simulink model "02-07-2026"  (R2025b)
settings: Solver=ode5  StartTime=0.0  StopTime=150  FixedStep=1/3200  RelTol=1e-3
model workspace (MAT data in the model file):
  mass = 7
  radius = 333
libraries: simulink x5, simulink_extras x4, eeGeneralControl x2
settings Model: Creator=Fabian  LastModifiedBy=fabia

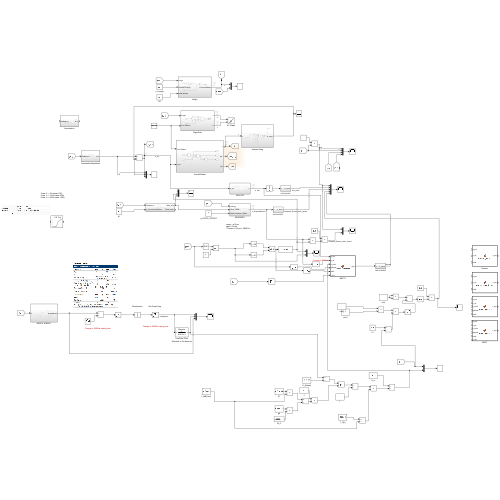
[thumbnail: Simulink's stored preview of the top-level diagram]
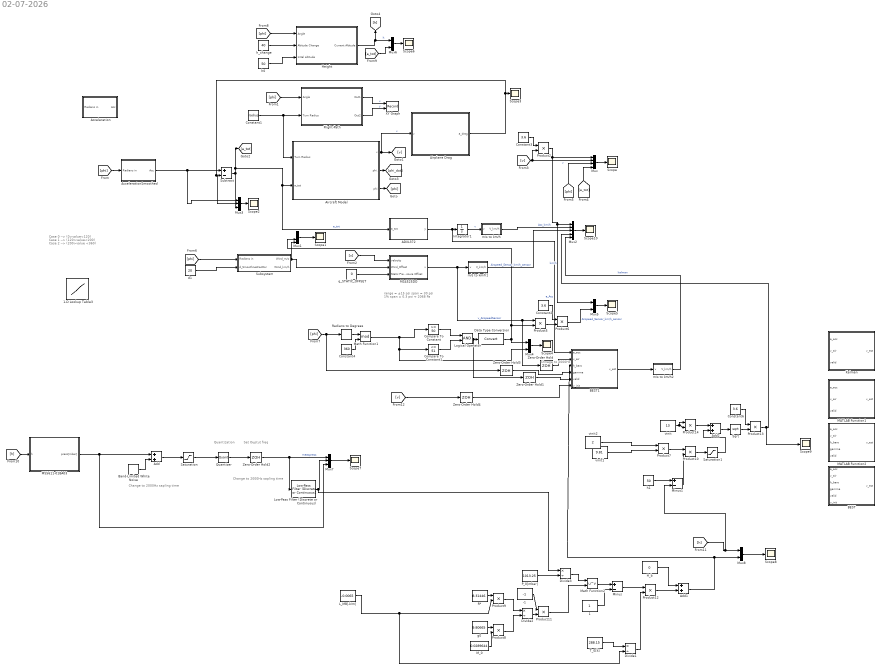
== system 02-07-2026 ==
  note: Change to 2000Hz sapling time
  note: Chnage to 2000Hz
  note: range = ±15 psi
      | span = 30 psi
      | 1% span = 0.3 psi ≈ 2068 Pa
  note: Case 0 --> (0>value<120)
      | Case 1 --> (120>value<200)
      | Case 2 --> (200>value <360)
  note: Set Ouptut freq
  note: Quantization
  note: Change to 2000Hz sapling time
  -1 : Constant  Value=-1
  1 : Constant
  1-D Lookup Table3 : Lookup_n-D  NumberOfTableDimensions=1  BreakpointsForDimension1=[0 110 130 190 210 360]  Table=[30 20 30 60 90 120]  InternalRulePriority=Speed  RndMeth=Simplest
  ADXL372 : Subsystem
  Acceleration : Subsystem
  AccelerationSmoothed : Subsystem
  Add : Sum
  Add1 : Sum
  Add2 : Sum
  Aircraft Model : Subsystem
  Airplane Drag : Subsystem
  BEST : MATLAB Function  TreatAsAtomicUnit=on
  BEST1 : MATLAB Function  TreatAsAtomicUnit=on
  Band-Limited White Noise : simulink/Sources/Band-Limited White Noise  Cov=(0.065)^2 * (1/2000)  Ts=1/3200  seed=[23341]
  Compare To Constant : simulink/Logic and Bit Operations/Compare To Constant  relop=>=  const=50  OutDataTypeStr=boolean
  Compare To Constant1 : simulink/Logic and Bit Operations/Compare To Constant  relop=<=  const=51  OutDataTypeStr=boolean
  Constant1 : Constant  Value=radius
  Constant2 : Constant  Value=3.6
  Constant3 : Constant  Value=3.6
  Constant4 : Constant  Value=360
  Constant6 : Constant  Value=3.6
  Data Type Conversion : DataTypeConversion  SaturateOnIntegerOverflow=off  RndMeth=Floor
  Divide1 : Product  Inputs=*/
  Divide2 : Product  Inputs=*/
  Divide3 : Product  Inputs=*/
  Flight-Path : Subsystem
  H_b : Constant  Value=0
  Height : Subsystem
  Integrator1 : Integrator  InitialCondition=13
  Kalman : MATLAB Function  TreatAsAtomicUnit=on
  L_MB[-k/m] : Constant  Value=-0.0065
  Logical Operator : Logic  AllPortsSameDT=off  OutDataTypeStr=fixdt(1,16)
  Low-Pass Filter (Discrete or Continuous) : eeGeneralControl/Low-Pass Filter (Discrete or Continuous)  K=1  T=0.021  B=inf  A=-inf  init_option=Inherited from block input  x0=0  Ts=-1
  MATLAB Function1 : MATLAB Function  TreatAsAtomicUnit=on
  MATLAB Function2 : MATLAB Function  TreatAsAtomicUnit=on
  MS4525DO : Subsystem
  "MS5611-01BA03 " : Subsystem
  M_0 : Constant  Value=0.0289644
  Math Function1 : Math  Operator=mod
  Math Function2 : Math  Operator=pow
  Minus : Sum  Inputs=+-
  Minus1 : Sum  Inputs=+-
  Mux : Mux
  Mux1 : Mux
  Mux2 : Mux  Inputs=5
  Mux3 : Mux  Inputs=3
  Mux{4..6,8} (4 alike) : Mux  Inputs=2
  Mux7 : Mux  Inputs=3
  P_0[mbar] : Constant  Value=1013.25
  Product{2,5..14} (11 alike) : Product
  Quantizer : Quantizer  QuantizationInterval=(1200-10)/(2^24)
  R* : Constant  Value=8.31446
  Radians to Degrees : simulink_extras/Transformations/Radians to Degrees
  Saturation : Saturate  UpperLimit=1200  LowerLimit=10
  Saturation1 : Saturate  UpperLimit=inf  LowerLimit=0.1
  Scope{,1..10} (11 alike) : Scope
      Scope settings: ActiveDisplayYMinimum=-135.5578997044986  ActiveDisplayYMaximum=1137.6664983393619
      Scope1 settings: ActiveDisplayYMinimum=-14.999999155382156  ActiveDisplayYMaximum=134.99999239843945  DataLoggingVariableName=ScopeData2
      Scope10 settings: ActiveDisplayYMinimum=-69.890870936461468  ActiveDisplayYMaximum=1097.0178384281537  DataLoggingVariableName=ScopeData11
      Scope2 settings: ActiveDisplayYMinimum=-39.208466924616559  ActiveDisplayYMaximum=63.33696033694325  DataLoggingVariableName=ScopeData3
      Scope3 settings: ActiveDisplayYMinimum=-3.5843354434410593  ActiveDisplayYMaximum=33.486381490969542  DataLoggingVariableName=ScopeData6
      Scope4 settings: ActiveDisplayYMinimum=-31.576019805247327  ActiveDisplayYMaximum=399.38392905519919  DataLoggingVariableName=ScopeData9
      Scope5 settings: ActiveDisplayYMinimum=189.29544667943134  ActiveDisplayYMaximum=704.92209117020684  DataLoggingVariableName=ScopeData12
      Scope6 settings: ActiveDisplayYMinimum=-31.394100237137991  ActiveDisplayYMaximum=92.400581276019  DataLoggingVariableName=ScopeData13
      Scope7 settings: ActiveDisplayYMinimum=1004.7404966647082  ActiveDisplayYMaximum=1013.7440475042908  DataLoggingVariableName=ScopeData14
      Scope8 settings: ActiveDisplayYMinimum=85.0381751510035  ActiveDisplayYMaximum=91.4462483318631  DataLoggingVariableName=ScopeData15
      Scope9 settings: ActiveDisplayYMinimum=38.767930934422381  ActiveDisplayYMaximum=119.22706265224174  DataLoggingVariableName=ScopeData16
  Sqrt : Sqrt
  Subsystem : Subsystem
  Subtract : Sum  Inputs=+-
  T_0[k] : Constant  Value=288.15
  XY Graph : Record  NumPorts=2.0  FileSettingsInternal="{\"entries\":[{\"content\":{\"excelSettings\":{\"content\":{},\"type\":\"Streamout.ExcelSettings\"},\"parquetSettings\":{\"content\":{},\"type\":\"Streamout.ParquetSettings\"}},\"type\":\"Streamout.FileSettingStorage\",\"uuid\":\"\"}],\"packageUris\":[\"http:\\/\\/schema.mathworks.com\\/mf0\\/streamout_blocks\\/R2020a\"],\"version\":\"1.0\"}"  FrameSettings=[0, 0]  Layout=[1 1]  SignalsInternal="{\"entries\":[{\"content\":{\"signals\":[{\"content\":{\"blockPath\":[],\"dimensions\":[1],\"domain\":\"\",\"lineColor\":\"#a2142f\",\"plots\":[ 1 ],\"port\":1,\"sid\":[\"\"],\"signalID\":1,\"signalName\":\"x\"},\"type\":\"RecordBlkView.Signal\",\"uuid\":\"\"},{\"content\":{\"blockPath\":[],\"dimensions\":[1],\"domain\":\"\",\"lineColor\":\"#139fff\",\"plots\":[ 1 ],\"port\":2,\"sid\":[\"\"],\"signalID\":2,\"signalName\":\"y\"},\"type\":\"RecordBlkView.Signal\",\"uuid\":\"\"}]},\"type\":\"RecordBlkView.InputSignals\",\"uuid\":\"\"}],\"packageUris\":[\"http:\\/\\/schema.mathworks.com\\/mf0\\/streamout_blocks\\/R2020a\"],\"version\":\"1.0\"}"  VisualizationBindings="{\"xyplotplugin\":{\"info\":[{\"series\":[{\"bindingParametersList\":[{\"parameter\":\"X-Axis\",\"signalID\":1,\"signalName\":\"x\"},{\"parameter\":\"Y-Axis\",\"signalID\":2,\"signalName\":\"y\"}],\"seriesID\":0}],\"subplotID\":1}]}}"  CompatibilityTag=XY
  Zero-Order Hold{,1..4} (5 alike) : ZeroOrderHold  SampleTime=1/3200
  d1 : Constant  Value=20
  g0 : Constant  Value=9.80665
  h0 : Constant  Value=50
  h1 : Constant  Value=50
  h_change : Constant  Value=40
  m/s to km/h : Subsystem
  m/s to km/h1 : Subsystem
  m/s to km/h2 : Subsystem
  q_STATIC_OFFSET : Constant  Value=0
  vinit : Constant  Value=13
  vinit1 : Constant  Value=9.81
  vinit2 : Constant  Value=2
  wires:
  Subtract/1 -> [a_tot], ADXL372/1(a_tot), Aircraft Model/2(a_tot), Mux3/3  "a_tot"
  Constant1/1 -> Flight-Path/2(Turn Radius), Aircraft Model/1(Turn Radius)
  Product2/1 -> Mux2/1, Mux5/1, Mux/1  "km/h"
  Mux2/1 -> Scope10/1
  ADXL372/1(y) -> BEST1/1(a_acc), Integrator1/1  "a_Acc"
  [phi] -> AccelerationSmoothed/1(Radians in)
  m/s to km/h1/1(V_km/h) -> Mux2/3  "Airspeed_Sensor_km/h_sensor"
  [v] -> MS4525DO/1(velocity)
  q_STATIC_OFFSET/1 -> MS4525DO/3(Static Pressure Offset)
  MS4525DO/1(v) -> m/s to km/h1/1(v), Zero-Order Hold/1, Product5/1  "v_AirspeedSensor"
  [phi] -> Flight-Path/1(Angle)
  Flight-Path/1(Out1) -> XY Graph/1  "x"
  Flight-Path/2(Out2) -> XY Graph/2  "y"
  [v] -> Product2/2, Mux/2  "v"
  [a_tot] -> Mux/4
  [phi] -> Mux/3
  Aircraft Model/1(v) -> Airplane Drag/1(v), [v]  "v"
  Aircraft Model/2(phi.) -> [phi_dot]
  Aircraft Model/3(phi) -> [phi]
  Constant3/1 -> Product2/1
  Mux/1 -> Scope/1
  Mux1/1 -> Scope1/1
  Mux3/1 -> Scope2/1
  [phi] -> Subsystem/1(Radians in)
  d1/1 -> Subsystem/2(d_SmoothnesFacttor)
  Subsystem/1(Wind_m/s) -> Mux1/4, MS4525DO/2(Wind_Offset)
  AccelerationSmoothed/1(Acc) -> Mux3/1, Subtract/1
  [phi] -> Zero-Order Hold3/1, Radians to Degrees/1
  Radians to Degrees/1 -> Math Function1/1
  Constant4/1 -> Math Function1/2
  Math Function1/1 -> Compare To Constant/1, Compare To Constant1/1, Mux4/2
  Compare To Constant/1 -> Logical Operator/1
  Compare To Constant1/1 -> Logical Operator/2
  Logical Operator/1 -> Zero-Order Hold1/1, Data Type Conversion/1
  Mux4/1 -> Scope4/1
  Data Type Conversion/1 -> Mux1/3, Product5/2, Mux4/1
  Mux5/1 -> Scope5/1
  Constant2/1 -> Product6/1
  Product5/1 -> Product6/2
  Product6/1 -> Mux5/2  "Airspeed_Sensor_km/h_sensor"
  Zero-Order Hold/1 -> BEST1/2(v_air)
  Zero-Order Hold1/1 -> BEST1/5(valid)
  h0/1 -> Height/3(Inital altitude)
  h_change/1 -> Height/2(Altitude Change)
  [phi] -> Height/1(Angle)
  Mux6/1 -> Scope6/1
  Height/1(Current Altitude) -> [h], Mux6/1  "h"
  [a_tot] -> Mux6/2
  "MS5611-01BA03 "/1(press[mbar]) -> Add/1, Mux7/3
  [h] -> "MS5611-01BA03 "/1(h)
  Band-Limited White Noise/1 -> Add/2
  Quantizer/1 -> Zero-Order Hold2/1
  Saturation/1 -> Quantizer/1
  Add/1 -> Saturation/1
  Zero-Order Hold2/1 -> Low-Pass Filter (Discrete or Continuous)/1, Mux7/1  "measpress"
  g0/1 -> Product8/1
  M_0/1 -> Product8/2
  L_MB[-k/m]/1 -> Divide1/2, Product9/2
  R*/1 -> Product9/1
  Mux8/1 -> Scope8/1
  [h] -> Minus1/2, Mux8/1
  Mux7/1 -> Scope7/1
  Product9/1 -> Divide2/1
  Product8/1 -> Divide2/2
  Divide2/1 -> Product11/2
  -1/1 -> Product11/1
  Product11/1 -> Math Function2/2
  Divide3/1 -> Math Function2/1
  P_0[mbar]/1 -> Divide3/2
  1/1 -> Minus/2
  Math Function2/1 -> Minus/1
  Minus/1 -> Product12/1
  T_0[k]/1 -> Divide1/1
  Divide1/1 -> Product12/2
  Product12/1 -> Add1/2
  H_b/1 -> Add1/1
  Add1/1 -> BEST1/3(h_baro), Mux8/2
  Low-Pass Filter (Discrete or Continuous)/1 -> Divide3/1, Mux7/2
  Zero-Order Hold3/1 -> BEST1/4(gamma)
  [v] -> Zero-Order Hold4/1
  Zero-Order Hold4/1 -> BEST1/6(v_init)
  vinit1/1 -> Product7/2
  vinit2/1 -> Product7/1
  h1/1 -> Minus1/1
  Product7/1 -> Product10/1
  Minus1/1 -> Product10/2
  Add2/1 -> Sqrt/1
  m/s to km/h2/1(V_km/h) -> Mux2/5  "kalman"
  Sqrt/1 -> Product13/2
  Constant6/1 -> Product13/1
  Product13/1 -> Scope9/1, Mux2/4
  vinit/1 -> Product14/1, Product14/2
  Product14/1 -> Add2/1
  Saturation1/1 -> Add2/2
  Product10/1 -> Saturation1/1
  Airplane Drag/1(a_drag) -> Mux3/2, Subtract/2, Scope3/1
  Integrator1/1 -> m/s to km/h/1(v)  "v"
  m/s to km/h/1(V_km/h) -> Mux2/2  "Acc_km/h"
  BEST1/1(v_est) -> m/s to km/h2/1(v)

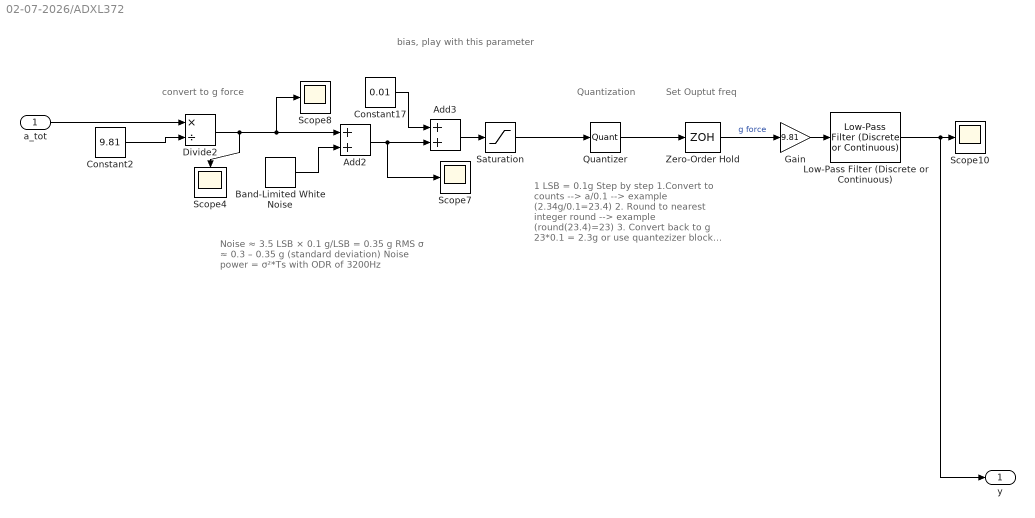
== system 02-07-2026/ADXL372 ==
  note: convert to g force
  note: Noise ≈ 3.5 LSB × 0.1 g/LSB = 0.35 g RMS
      | σ ≈ 0.3 – 0.35 g (standard deviation)
      | Noise power = σ²*Ts
      | with ODR of 3200Hz
  note: bias, play with this parameter
  note: Quantization
  note: 1 LSB = 0.1g
      | Step by step
      |
      | 1.Convert to counts
      | --> a/0.1 --> example (2.34g/0.1=23.4)
      | 2. Round to nearest integer
      | round --> example (round(23.4)=23)
      | 3. Convert back to g
      | 23*0.1 = 2.3g
      |
      | or use quantezizer block with 0.1
  note: Set Ouptut freq
  a_tot : Inport
  Add2 : Sum
  Add3 : Sum
  Band-Limited White Noise : simulink/Sources/Band-Limited White Noise  Cov=((0.35)^2)*(1/3200)  Ts=1/3200  seed=[23341]
  Constant17 : Constant  Value=0.01
  Constant2 : Constant  Value=9.81
  Divide2 : Product  Inputs=*/
  Gain : Gain  Gain=9.81
  Low-Pass Filter (Discrete or Continuous) : eeGeneralControl/Low-Pass Filter (Discrete or Continuous)  K=1  T=1/(2*pi*10)  B=inf  A=-inf  init_option=Inherited from block input  x0=0  Ts=1/3200
  Quantizer : Quantizer  QuantizationInterval=0.1
  Saturation : Saturate  UpperLimit=200  LowerLimit=-200
  Scope{4,7..8,10} (4 alike) : Scope
      Scope10 settings: ActiveDisplayYMinimum=-5.375623541068566  ActiveDisplayYMaximum=9.3751831580889746  DataLoggingVariableName=ScopeData10
      Scope4 settings: ActiveDisplayYMinimum=-8.7987661112898756  ActiveDisplayYMaximum=16.470735842466532  DataLoggingVariableName=ScopeData4
      Scope7 settings: ActiveDisplayYMinimum=-2.1194574766866134  ActiveDisplayYMaximum=2.6082539117818122  DataLoggingVariableName=ScopeData7
      Scope8 settings: ActiveDisplayYMinimum=-0.3058103975535168  ActiveDisplayYMaximum=0.71355759429153931  DataLoggingVariableName=ScopeData8
  Zero-Order Hold : ZeroOrderHold  SampleTime=1/3200
  y : Outport
  wires:
  Constant2/1 -> Divide2/2
  Add3/1 -> Saturation/1
  Saturation/1 -> Quantizer/1
  Divide2/1 -> Add2/1, Scope8/1, Scope4/1
  Gain/1 -> Low-Pass Filter (Discrete or Continuous)/1
  Add2/1 -> Scope7/1, Add3/2
  Constant17/1 -> Add3/1
  Band-Limited White Noise/1 -> Add2/2
  Quantizer/1 -> Zero-Order Hold/1
  Zero-Order Hold/1 -> Gain/1  "g force"
  Low-Pass Filter (Discrete or Continuous)/1 -> y/1, Scope10/1
  a_tot/1 -> Divide2/1

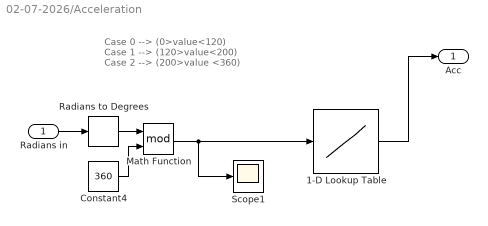
== system 02-07-2026/Acceleration ==
  note: Case 0 --> (0>value<120)
      | Case 1 --> (120>value<200)
      | Case 2 --> (200>value <360)
  Radians in : Inport
  1-D Lookup Table : Lookup_n-D  NumberOfTableDimensions=1  BreakpointsForDimension1=[0 120 130 190 210 360]  Table=[-3 -3 6 6 4 4]  InterpMethod=Linear Lagrange  InternalRulePriority=Speed  RndMeth=Simplest
  Constant4 : Constant  Value=360
  Math Function : Math  Operator=mod
  Radians to Degrees : simulink_extras/Transformations/Radians to Degrees
  Scope1 : Scope
      settings: ActiveDisplayYMinimum=2.9529948597935629  ActiveDisplayYMaximum=755.41634315848091
  Acc : Outport
  wires:
  Radians to Degrees/1 -> Math Function/1
  Constant4/1 -> Math Function/2
  Math Function/1 -> Scope1/1, 1-D Lookup Table/1
  Radians in/1 -> Radians to Degrees/1
  1-D Lookup Table/1 -> Acc/1

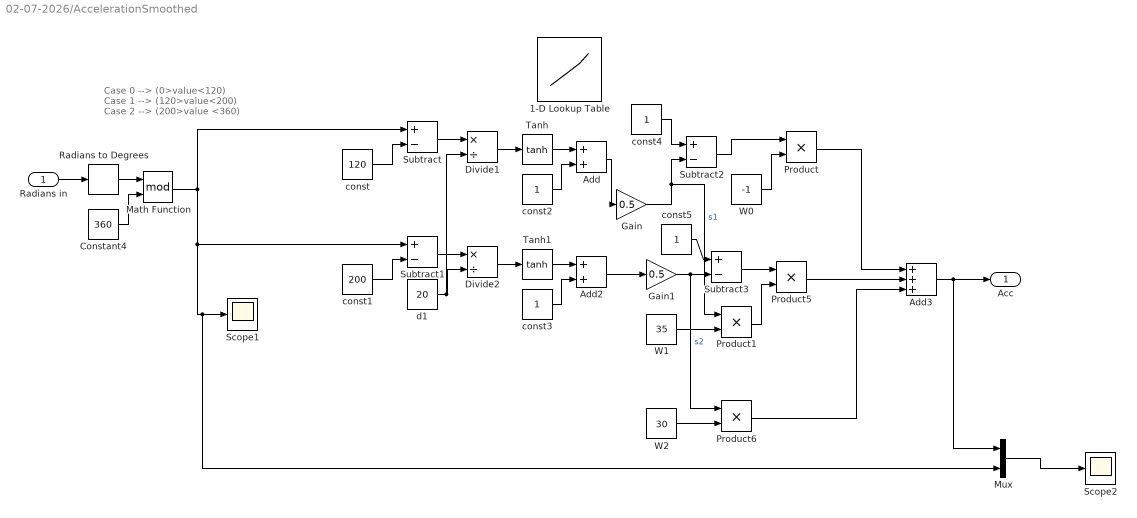
== system 02-07-2026/AccelerationSmoothed ==
  note: Case 0 --> (0>value<120)
      | Case 1 --> (120>value<200)
      | Case 2 --> (200>value <360)
  Radians in : Inport
  1-D Lookup Table : Lookup_n-D  NumberOfTableDimensions=1  BreakpointsForDimension1=[0 110 130 190 210 360]  Table=[-3 -3 6 6 4 4]  InterpMethod=Linear Lagrange  InternalRulePriority=Speed  RndMeth=Simplest
  Add : Sum
  Add2 : Sum
  Add3 : Sum  Inputs=+++
  Constant4 : Constant  Value=360
  Divide1 : Product  Inputs=*/
  Divide2 : Product  Inputs=*/
  Gain : Gain  Gain=0.5
  Gain1 : Gain  Gain=0.5
  Math Function : Math  Operator=mod
  Mux : Mux  Inputs=2
  Product{,1,5..6} (4 alike) : Product
  Radians to Degrees : simulink_extras/Transformations/Radians to Degrees
  Scope1 : Scope
      settings: ActiveDisplayYMinimum=-47.332509505790171  ActiveDisplayYMaximum=913.02258838484045
  Scope2 : Scope
      settings: ActiveDisplayYMinimum=-16.733117928341755  ActiveDisplayYMaximum=372.27391286785394  DataLoggingVariableName=ScopeData5
  Subtract{,1..3} (4 alike) : Sum  Inputs=+-
  Tanh : Trigonometry  Operator=tanh
  Tanh1 : Trigonometry  Operator=tanh
  W0 : Constant  Value=-1
  W1 : Constant  Value=35
  W2 : Constant  Value=30
  const : Constant  Value=120
  const1 : Constant  Value=200
  const{2..5} (4 alike) : Constant
  d1 : Constant  Value=20
  Acc : Outport
  wires:
  Radians to Degrees/1 -> Math Function/1
  Constant4/1 -> Math Function/2
  Radians in/1 -> Radians to Degrees/1
  W1/1 -> Product1/2
  W0/1 -> Product/2
  Math Function/1 -> Subtract1/1, Mux/2, Scope1/1, Subtract/1
  const4/1 -> Subtract2/1
  Tanh/1 -> Add/1
  const2/1 -> Add/2
  Add/1 -> Gain/1
  Product1/1 -> Product5/2
  Tanh1/1 -> Add2/1
  Subtract3/1 -> Product5/1
  Product6/1 -> Add3/3
  Subtract2/1 -> Product/1
  Subtract/1 -> Divide1/1
  const3/1 -> Add2/2
  Divide1/1 -> Tanh/1
  const/1 -> Subtract/2
  const1/1 -> Subtract1/2
  Subtract1/1 -> Divide2/1
  d1/1 -> Divide1/2, Divide2/2
  const5/1 -> Subtract3/1
  Gain1/1 -> Product6/1, Subtract3/2  "s2"
  Product5/1 -> Add3/2
  Add2/1 -> Gain1/1
  Gain/1 -> Subtract2/2, Product1/1  "s1"
  Divide2/1 -> Tanh1/1
  Product/1 -> Add3/1
  W2/1 -> Product6/2
  Add3/1 -> Mux/1, Acc/1
  Mux/1 -> Scope2/1

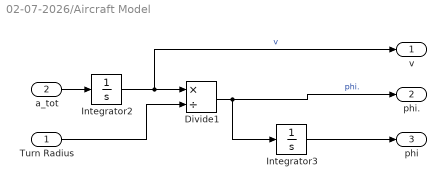
== system 02-07-2026/Aircraft Model ==
  Turn Radius : Inport
  a_tot : Inport  Port=2
  Divide1 : Product  Inputs=*/
  Integrator2 : Integrator  InitialCondition=13
  Integrator3 : Integrator  InitialCondition=pi
  v : Outport
  phi. : Outport  Port=2
  phi : Outport  Port=3
  wires:
  Divide1/1 -> phi./1, Integrator3/1  "phi."
  Integrator3/1 -> phi/1
  Integrator2/1 -> v/1, Divide1/1  "v"
  Turn Radius/1 -> Divide1/2
  a_tot/1 -> Integrator2/1

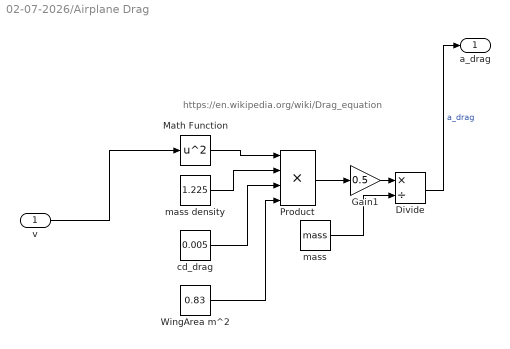
== system 02-07-2026/Airplane Drag ==
  note: https://en.wikipedia.org/wiki/Drag_equation
  v : Inport
  Divide : Product  Inputs=*/
  Gain1 : Gain  Gain=0.5
  Math Function : Math  Operator=square
  Product : Product  Inputs=4
  WingArea m^2 : Constant  Value=0.83
  cd_drag : Constant  Value=0.005
  mass : Constant  Value=mass
  mass density : Constant  Value=1.225
  a_drag : Outport
  wires:
  mass/1 -> Divide/2
  mass density/1 -> Product/2
  Divide/1 -> a_drag/1  "a_drag"
  Math Function/1 -> Product/1
  cd_drag/1 -> Product/3
  Gain1/1 -> Divide/1
  WingArea m^2/1 -> Product/4
  Product/1 -> Gain1/1
  v/1 -> Math Function/1

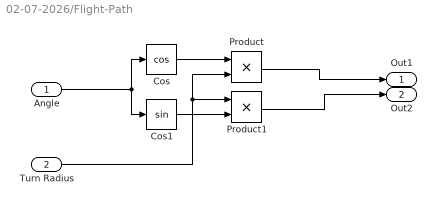
== system 02-07-2026/Flight-Path ==
  Angle : Inport
  Turn Radius : Inport  Port=2
  Cos : Trigonometry  Operator=cos
  Cos1 : Trigonometry
  Product : Product
  Product1 : Product
  Out1 : Outport
  Out2 : Outport  Port=2
  wires:
  Cos1/1 -> Product1/2
  Turn Radius/1 -> Product/2, Product1/1
  Angle/1 -> Cos1/1, Cos/1
  Cos/1 -> Product/1
  Product1/1 -> Out2/1
  Product/1 -> Out1/1

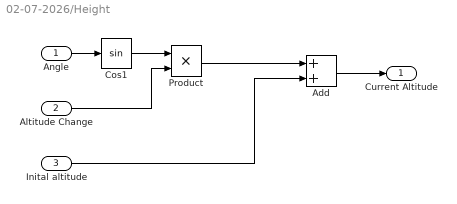
== system 02-07-2026/Height ==
  Angle : Inport
  Altitude Change : Inport  Port=2
  Inital altitude : Inport  Port=3
  Add : Sum
  Cos1 : Trigonometry
  Product : Product
  Current Altitude : Outport
  wires:
  Angle/1 -> Cos1/1
  Inital altitude/1 -> Add/2
  Altitude Change/1 -> Product/2
  Cos1/1 -> Product/1
  Product/1 -> Add/1
  Add/1 -> Current Altitude/1

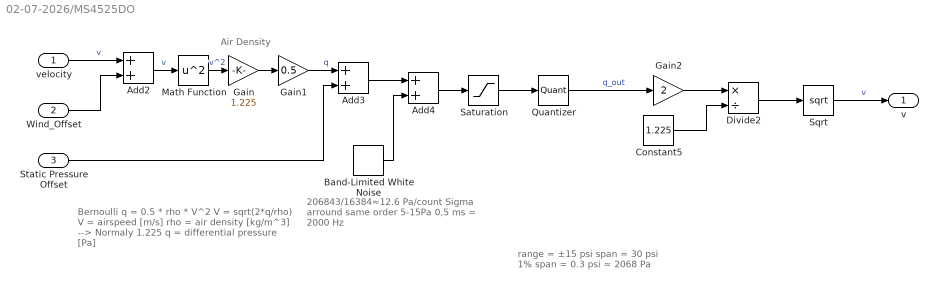
== system 02-07-2026/MS4525DO ==
  note: Bernoulli
      | q = 0.5 * rho * V^2
      | V = sqrt(2*q/rho)
      |
      | V = airspeed [m/s]
      | rho = air density [kg/m^3] --> Normaly 1.225
      | q = differential pressure [Pa]
  note: Air Density
  note: 206843/16384​≈12.6 Pa/count
      | Sigma arround same order 5-15Pa
      |
      | 0,5 ms = 2000 Hz
  note: range = ±15 psi
      | span = 30 psi
      | 1% span = 0.3 psi ≈ 2068 Pa
  velocity : Inport
  Wind_Offset : Inport  Port=2
  Static Pressure Offset : Inport  Port=3
  Add2 : Sum
  Add3 : Sum
  Add4 : Sum
  Band-Limited White Noise : simulink/Sources/Band-Limited White Noise  Cov=((10)^2)*(1/3200)  Ts=1/3200  seed=[23341]
  Constant5 : Constant  Value=1.225
  Divide2 : Product  Inputs=*/
  Gain : Gain  Gain=1.225
  Gain1 : Gain  Gain=0.5
  Gain2 : Gain  Gain=2
  Math Function : Math  Operator=square
  Quantizer : Quantizer  QuantizationInterval=12.6
  Saturation : Saturate  UpperLimit=103421  LowerLimit=-103421
  Sqrt : Sqrt
  v : Outport
  wires:
  Add3/1 -> Add4/1
  Divide2/1 -> Sqrt/1
  Add2/1 -> Math Function/1  "v"
  Saturation/1 -> Quantizer/1
  Math Function/1 -> Gain/1  "v^2"
  Gain/1 -> Gain1/1
  Gain1/1 -> Add3/1  "q"
  Add4/1 -> Saturation/1
  Gain2/1 -> Divide2/1
  Wind_Offset/1 -> Add2/2
  Constant5/1 -> Divide2/2
  Quantizer/1 -> Gain2/1  "q_out"
  Band-Limited White Noise/1 -> Add4/2
  velocity/1 -> Add2/1  "v"
  Static Pressure Offset/1 -> Add3/2
  Sqrt/1 -> v/1  "v"

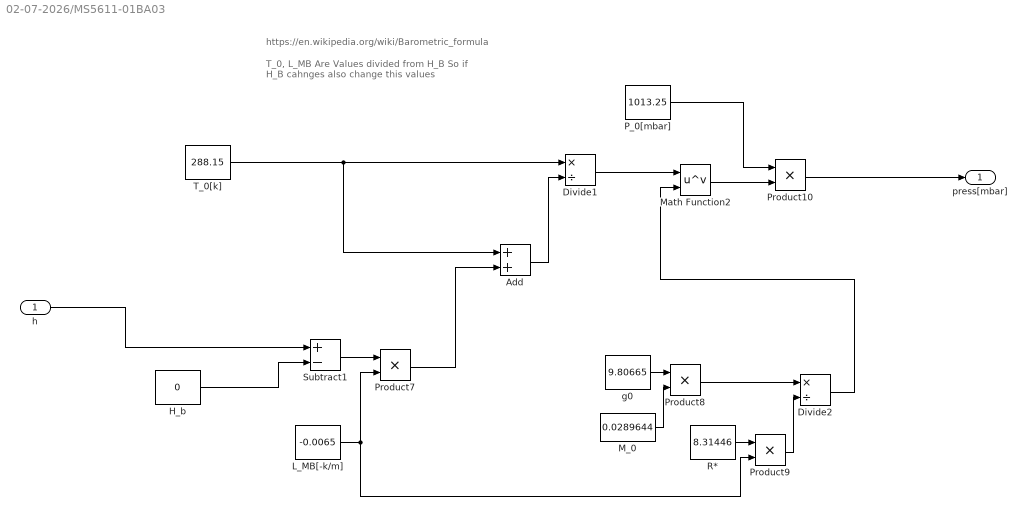
== system 02-07-2026/MS5611-01BA03  ==
  note: https://en.wikipedia.org/wiki/Barometric_formula
  note: T_0, L_MB
      | Are Values divided from H_B
      | So if H_B cahnges also change this values
  h : Inport
  Add : Sum
  Divide1 : Product  Inputs=*/
  Divide2 : Product  Inputs=*/
  H_b : Constant  Value=0
  L_MB[-k/m] : Constant  Value=-0.0065
  M_0 : Constant  Value=0.0289644
  Math Function2 : Math  Operator=pow
  P_0[mbar] : Constant  Value=1013.25
  Product{7..10} (4 alike) : Product
  R* : Constant  Value=8.31446
  Subtract1 : Sum  Inputs=+-
  T_0[k] : Constant  Value=288.15
  g0 : Constant  Value=9.80665
  press[mbar] : Outport
  wires:
  R*/1 -> Product9/1
  L_MB[-k/m]/1 -> Product9/2, Product7/2
  Product9/1 -> Divide2/2
  g0/1 -> Product8/1
  h/1 -> Subtract1/1
  M_0/1 -> Product8/2
  T_0[k]/1 -> Add/1, Divide1/1
  Add/1 -> Divide1/2
  Subtract1/1 -> Product7/1
  P_0[mbar]/1 -> Product10/1
  Math Function2/1 -> Product10/2
  Product7/1 -> Add/2
  Divide2/1 -> Math Function2/2
  H_b/1 -> Subtract1/2
  Product8/1 -> Divide2/1
  Divide1/1 -> Math Function2/1
  Product10/1 -> press[mbar]/1

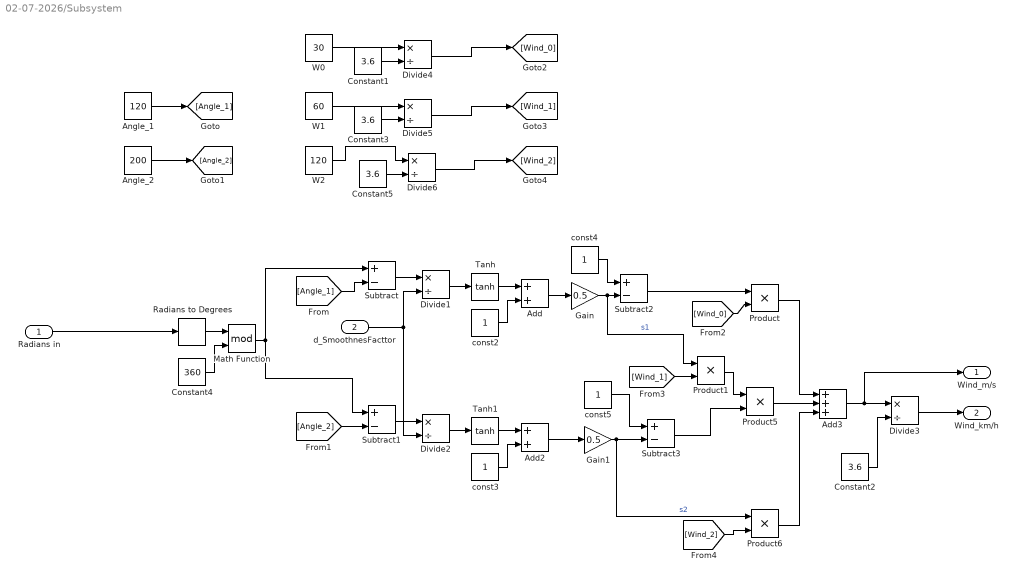
== system 02-07-2026/Subsystem ==
  Radians in : Inport
  d_SmoothnesFacttor : Inport  Port=2
  Add : Sum
  Add2 : Sum
  Add3 : Sum  Inputs=+++
  Angle_1 : Constant  Value=120
  Angle_2 : Constant  Value=200
  Constant{1..3,5} (4 alike) : Constant  Value=3.6
  Constant4 : Constant  Value=360
  Divide{1..6} (6 alike) : Product  Inputs=*/
  Gain : Gain  Gain=0.5
  Gain1 : Gain  Gain=0.5
  Math Function : Math  Operator=mod
  Product{,1,5..6} (4 alike) : Product
  Radians to Degrees : simulink_extras/Transformations/Radians to Degrees
  Subtract{,1..3} (4 alike) : Sum  Inputs=+-
  Tanh : Trigonometry  Operator=tanh
  Tanh1 : Trigonometry  Operator=tanh
  W0 : Constant  Value=30
  W1 : Constant  Value=60
  W2 : Constant  Value=120
  const{2..5} (4 alike) : Constant
  Wind_m/s : Outport
  Wind_km/h : Outport  Port=2
  wires:
  Math Function/1 -> Subtract/1, Subtract1/1
  Divide3/1 -> Wind_km/h/1
  Subtract1/1 -> Divide2/1
  Gain/1 -> Product1/1, Subtract2/2  "s1"
  Divide2/1 -> Tanh1/1
  Gain1/1 -> Subtract3/2, Product6/1  "s2"
  Product6/1 -> Add3/3
  Subtract2/1 -> Product/1
  Divide1/1 -> Tanh/1
  const2/1 -> Add/2
  Constant2/1 -> Divide3/2
  Subtract/1 -> Divide1/1
  const3/1 -> Add2/2
  Tanh1/1 -> Add2/1
  Product/1 -> Add3/1
  Add/1 -> Gain/1
  Add3/1 -> Wind_m/s/1, Divide3/1
  Tanh/1 -> Add/1
  d_SmoothnesFacttor/1 -> Divide2/2, Divide1/2
  Radians to Degrees/1 -> Math Function/1
  const4/1 -> Subtract2/1
  const5/1 -> Subtract3/1
  Product5/1 -> Add3/2
  Constant4/1 -> Math Function/2
  Add2/1 -> Gain1/1
  Radians in/1 -> Radians to Degrees/1
  Angle_1/1 -> [Angle_1]
  [Angle_1] -> Subtract/2
  Angle_2/1 -> [Angle_2]
  [Angle_2] -> Subtract1/2
  [Wind_0] -> Product/2
  [Wind_1] -> Product1/2
  Subtract3/1 -> Product5/2
  Product1/1 -> Product5/1
  [Wind_2] -> Product6/2
  Constant1/1 -> Divide4/2
  W0/1 -> Divide4/1
  Divide4/1 -> [Wind_0]
  W1/1 -> Divide5/1
  Constant3/1 -> Divide5/2
  Divide5/1 -> [Wind_1]
  Constant5/1 -> Divide6/2
  W2/1 -> Divide6/1
  Divide6/1 -> [Wind_2]

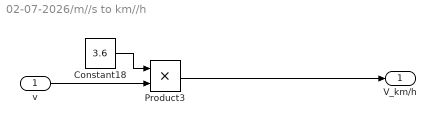
== system 02-07-2026/m//s to km//h ==
  v : Inport
  Constant18 : Constant  Value=3.6
  Product3 : Product
  V_km/h : Outport
  wires:
  Constant18/1 -> Product3/1
  Product3/1 -> V_km/h/1
  v/1 -> Product3/2

== system 02-07-2026/m//s to km//h1 ==
  v : Inport
  Constant18 : Constant  Value=3.6
  Product3 : Product
  V_km/h : Outport
  wires:
  Constant18/1 -> Product3/1
  Product3/1 -> V_km/h/1
  v/1 -> Product3/2

== system 02-07-2026/m//s to km//h2 ==
  v : Inport
  Constant18 : Constant  Value=3.6
  Product3 : Product
  V_km/h : Outport
  wires:
  Constant18/1 -> Product3/1
  Product3/1 -> V_km/h/1
  v/1 -> Product3/2

== matlab function 02-07-2026/Kalman ==
  data: a_acc input; v_est output; v_air input; valid input
function v_est = kalman_partial(a_acc, v_air, valid)
%#codegen

dt = 1/3200;     % set to your sample time
Q  = 1;         % tune
R  = 20;        % tune

persistent v P
if isempty(v)
    v = v_air;
    P = 100;
end

% Prediction from accelerometer
v_pred = v + a_acc * dt;
P_pred = P + Q;

if valid > 0.5
    % Correction only when airspeed is reliable
    K = P_pred / (P_pred + R);
    v = v_pred + K * (v_air - v_pred);
    P = (1 - K) * P_pred;
else
    % No airspeed correction
    v = v_pred;
    P = P_pred;
end

v_est = v;

== matlab function 02-07-2026/BEST1 ==
  data: a_acc input; v_est output; v_air input; h_baro input; gamma input; valid input; v_init input
function v_est = kalman_3sensor(a_acc, v_air, h_baro, gamma, valid, v_init)
%#codegen

dt = 1/3200;

Qv = 0.5;
Qh = 0.1;
Qb = 0.01;

R_air = 50000;
R_h   = 0.25;     % baro noise variance, e.g. 0.5m RMS -> 0.25

persistent x P
if isempty(x)
    x = [v_init; h_baro; 0];   % [speed; height; acc_bias]
    P = diag([100, 10, 1]);
end

v = x(1);
h = x(2);
b = x(3);

% Prediction
v_pred = v + (a_acc - b)*dt;
h_pred = h + v*sin(gamma)*dt;
b_pred = b;

x_pred = [v_pred; h_pred; b_pred];

P_pred = P + diag([Qv Qh Qb]);

x = x_pred;
P = P_pred;

% Airspeed update only in good zone
if valid > 0.5
    H_air = [1 0 0];
    K = P*H_air'/(H_air*P*H_air' + R_air);
    x = x + K*(v_air - H_air*x);
    P = (eye(3)-K*H_air)*P;
end

% Barometer height update
H_h = [0 1 0];
K = P*H_h'/(H_h*P*H_h' + R_h);
x = x + K*(h_baro - H_h*x);
P = (eye(3)-K*H_h)*P;

v_est = x(1);

== matlab function 02-07-2026/MATLAB Function1 ==
  data: a_acc input; v_est output; v_air input; valid input
function v_est = kalman_speed_bias(a_acc, v_air, valid)
%#codegen

dt = 1/3200;   % change to your sample time

Qv = 0.5;       % speed uncertainty
Qb = 0.01;    % airspeed bias can slowly change
R  = 400;      % airspeed noise

persistent x P
if isempty(x)
    x = [13; 0];      % [speed; airspeed_bias]
    P = diag([100, 100]);
end

% Prediction
A = [1 0;
     0 1];

B = [dt;
     0];

Q = diag([Qv Qb]);

x_pred = A*x + B*a_acc;
P_pred = A*P*A' + Q;

% Measurement: v_air = speed + bias
H = [1 1];

if valid > 0.5
    K = P_pred*H'/(H*P_pred*H' + R);
    x = x_pred + K*(v_air - H*x_pred);
    P = (eye(2) - K*H)*P_pred;
else
    x = x_pred;
    P = P_pred;
end

v_est = x(1);

== matlab function 02-07-2026/MATLAB Function2 ==
  data: a_acc input; v_est output; v_air input; h_baro input; gamma input; valid input
function v_est = kalman_3sensor(a_acc, v_air, h_baro, gamma, valid)
%#codegen

dt = 1/3200;

Qv = 0.5;
Qh = 0.1;
Qb = 0.001;

R_air = 10000;
R_h   = 0.25;     % baro noise variance, e.g. 0.5m RMS -> 0.25

persistent x P
if isempty(x)
    x = [v_air; h_baro; 0];   % [speed; height; acc_bias]
    P = diag([100, 10, 1]);
end

v = x(1);
h = x(2);
b = x(3);

% Prediction
v_pred = v + (a_acc - b)*dt;
h_pred = h + v*sin(gamma)*dt;
b_pred = b;

x_pred = [v_pred; h_pred; b_pred];

P_pred = P + diag([Qv Qh Qb]);

x = x_pred;
P = P_pred;

% Airspeed update only in good zone
if valid > 0.5
    H_air = [1 0 0];
    K = P*H_air'/(H_air*P*H_air' + R_air);
    x = x + K*(v_air - H_air*x);
    P = (eye(3)-K*H_air)*P;
end

% Barometer height update
H_h = [0 1 0];
K = P*H_h'/(H_h*P*H_h' + R_h);
x = x + K*(h_baro - H_h*x);
P = (eye(3)-K*H_h)*P;

v_est = x(1);

== matlab function 02-07-2026/BEST ==
  data: a_acc input; v_est output; v_air input; h_baro input; gamma input; valid input; v_init input
function v_est = kalman_3sensor(a_acc, v_air, h_baro, gamma, valid, v_init)
%#codegen

dt = 1/3200;

Qv = 0.5;
Qh = 0.1;
Qb = 0.01;

R_air = 50000;
R_h   = 0.25;     % baro noise variance, e.g. 0.5m RMS -> 0.25

persistent x P
if isempty(x)
    x = [v_init; h_baro; 0];   % [speed; height; acc_bias]
    P = diag([100, 10, 1]);
end

v = x(1);
h = x(2);
b = x(3);

% Prediction
v_pred = v + (a_acc - b)*dt;
h_pred = h + v*sin(gamma)*dt;
b_pred = b;

x_pred = [v_pred; h_pred; b_pred];

P_pred = P + diag([Qv Qh Qb]);

x = x_pred;
P = P_pred;

% Airspeed update only in good zone
if valid > 0.5
    H_air = [1 0 0];
    K = P*H_air'/(H_air*P*H_air' + R_air);
    x = x + K*(v_air - H_air*x);
    P = (eye(3)-K*H_air)*P;
end

% Barometer height update
H_h = [0 1 0];
K = P*H_h'/(H_h*P*H_h' + R_h);
x = x + K*(h_baro - H_h*x);
P = (eye(3)-K*H_h)*P;

v_est = x(1);
